simulink model "AreaCoverageTestHarness"  (R2016a)
settings: Solver=FixedStepDiscrete  StartTime=0.0  StopTime=6000  FixedStep=0.005  RelTol=1e-3
values from neighbouring files (symbols this model uses):
  BLOCK_SIZE = CAL_BLOCK_SIZE    [AreaCoverageCalib.m]    (also in room_V1.m = 20; room_V3.m = 20)
  EAST = 0    [AreaCoverageCalib.m]
  ERRVAL = 5    [AreaCoverageCalib.m]
  initXSim = 35    [AreaCoverageCalib.m]
  initYSim = 50    [AreaCoverageCalib.m]
  MAX_SPEED = 1000    [AreaCoverageCalib.m]
  MOTOR_HIGH = CAL_MOTOR_HIGH    [AreaCoverageCalib.m]
  MOTOR_LOW = CAL_MOTOR_LOW    [AreaCoverageCalib.m]
  NORTH = 270    [AreaCoverageCalib.m]
  PLOT_SAMPLE = 10    [AreaCoverageCalib.m]
  ROB_LENG = CAL_ROBO_LENG    [AreaCoverageCalib.m]
  ROB_WHEEL_R = .15    (= 0.15)    [AreaCoverageCalib.m]
  room = uint8(ones(side_size , side_size)*255)    [room_V1.m]    (also in room_V3.m)
  ROOM_SIDE_SIZE = CAL_ROOM_SIDE_SIZE    [AreaCoverageCalib.m]    (also in room_V1.m = 20; room_V3.m = 20)
  SAMPLE_TIME = 0.001    [AreaCoverageCalib.m]
  SOUTH = 90    [AreaCoverageCalib.m]
  STEP_SIZE = 5    [AreaCoverageCalib.m]
  WEST = 180    [AreaCoverageCalib.m]
undefined symbols (not defined in the file or in its folder): ROBO_LENG, sigbuilder_block
libraries: simulink x4
(part 1 of 2)
settings Model: Creator=oelkawok  LastModifiedBy=omaro

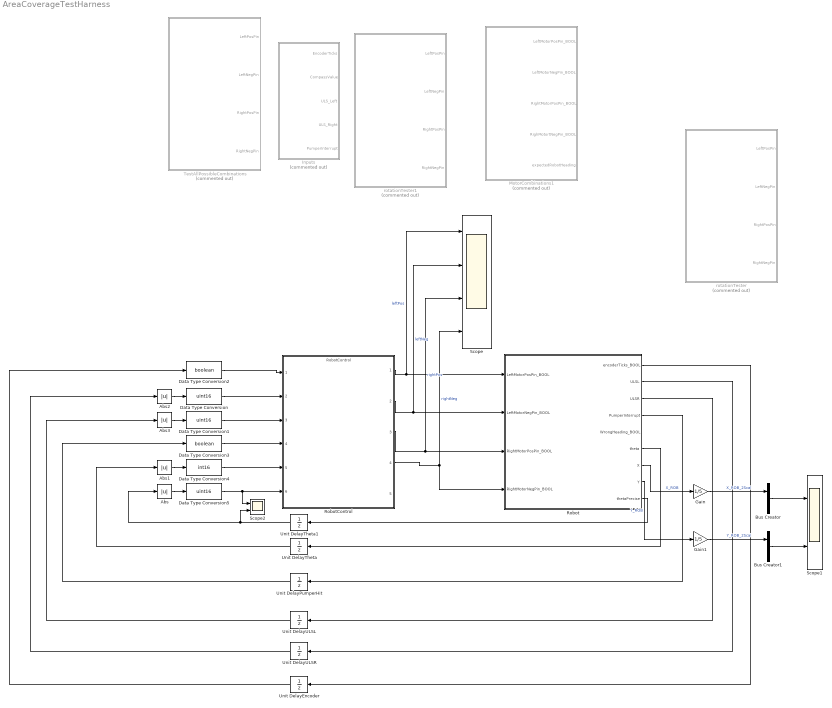
== system AreaCoverageTestHarness ==
  Abs{,1..3} (4 alike) : Abs
  Bus Creator : BusCreator  Inputs=2
  Bus Creator1 : BusCreator  Inputs=2
  Data Type Conversion : DataTypeConversion  OutDataTypeStr=uint16
  Data Type Conversion1 : DataTypeConversion  OutDataTypeStr=uint16
  Data Type Conversion2 : DataTypeConversion  OutDataTypeStr=boolean
  Data Type Conversion3 : DataTypeConversion  OutDataTypeStr=boolean
  Data Type Conversion4 : DataTypeConversion  OutDataTypeStr=int16
  Data Type Conversion5 : DataTypeConversion  OutDataTypeStr=uint16
  Gain : Gain  Gain=1/5  OutDataTypeStr=Inherit: Inherit via back propagation
  Gain1 : Gain  Gain=1/5  OutDataTypeStr=Inherit: Inherit via back propagation
  Inputs : Subsystem  Tag=STV Subsys  Commented=on  LoadFcn=sigbuilder_block('load');  StartFcn=sigbuilder_block('start');  StopFcn=sigbuilder_block('stop');  ClipboardFcn=sigbuilder_block('clipboard');  mask(Sigbuilder block){}
      mask help: Simulink:masks:SigbuilderBlock_MD
      mask init:
      | if ~strcmp(get_param(bdroot(gcbh),'SimulationStatus'),'stopped') tuvar = sigbuilder_block('maskInit'); end
      settings: CopyFcn=sigbuilder_block('copy');  DeleteFcn=sigbuilder_block('delete');  ModelCloseFcn=sigbuilder_block('modelClose');  PreSaveFcn=sigbuilder_block('preSave');  PauseFcn=sigbuilder_block('pause');  ContinueFcn=sigbuilder_block('continue');  NameChangeFcn=sigbuilder_block('namechange');  OpenFcn=sigbuilder_block('open',[211.2 103.8 550.8 400.2 ]);  CloseFcn=sigbuilder_block('close');
      mask Display: plot(0, 0, 100, 100,[2, 2, 32, 32, 2], [68, 8, 8, 68, 68],[32, 2], [38, 38], [32, 19, 2],[53, 60, 44], [32, 17, 17, 2],[16, 16, 31, 31]);txt = getActiveGroup(gcbh);text(2, 100, txt,'verticalAlignment', 'top');
  MotorCombinations1 : Subsystem  Commented=on
  Robot : Subsystem
  RobotControl : ModelReference  ModelNameDialog=RobotControl  SimulationMode=Normal  ModelReferenceVersion=1.370
  Scope : Scope  NumInputPorts=4
  Scope1 : Scope  NumInputPorts=2
  Scope2 : Scope  NumInputPorts=2
  TestAllPossibleCombinations : Subsystem  Tag=STV Subsys  Commented=on  LoadFcn=sigbuilder_block('load');  StartFcn=sigbuilder_block('start');  StopFcn=sigbuilder_block('stop');  ClipboardFcn=sigbuilder_block('clipboard');  mask(Sigbuilder block){}
      mask help: Simulink:masks:SigbuilderBlock_MD
      mask init:
      | if ~strcmp(get_param(bdroot(gcbh),'SimulationStatus'),'stopped') tuvar = sigbuilder_block('maskInit'); end
      settings: CopyFcn=sigbuilder_block('copy');  DeleteFcn=sigbuilder_block('delete');  ModelCloseFcn=sigbuilder_block('modelClose');  PreSaveFcn=sigbuilder_block('preSave');  PauseFcn=sigbuilder_block('pause');  ContinueFcn=sigbuilder_block('continue');  NameChangeFcn=sigbuilder_block('namechange');  OpenFcn=sigbuilder_block('open',[5.4 28.8 1141.2 525 ]);  CloseFcn=sigbuilder_block('close');
      mask Display: plot(0, 0, 100, 100,[2, 2, 32, 32, 2], [68, 8, 8, 68, 68],[32, 2], [38, 38], [32, 19, 2],[53, 60, 44], [32, 17, 17, 2],[16, 16, 31, 31]);txt = getActiveGroup(gcbh);text(2, 100, txt,'verticalAlignment', 'top');
  Unit DelayEncoder : UnitDelay  SampleTime=-1
  Unit DelayPumperHit : UnitDelay  SampleTime=-1
  Unit DelayTheta : UnitDelay  InitialCondition=NORTH  SampleTime=-1
      settings: AttributesFormatString=%<InitialCondition>
  Unit DelayTheta1 : UnitDelay  InitialCondition=NORTH*100  SampleTime=-1
      settings: AttributesFormatString=%<InitialCondition>
  Unit DelayULSL : UnitDelay  SampleTime=-1
  Unit DelayULSR : UnitDelay  SampleTime=-1
  rotationTester : Subsystem  Tag=STV Subsys  Commented=on  LoadFcn=sigbuilder_block('load');  StartFcn=sigbuilder_block('start');  StopFcn=sigbuilder_block('stop');  ClipboardFcn=sigbuilder_block('clipboard');  mask(Sigbuilder block){}
      mask help: Simulink:masks:SigbuilderBlock_MD
      mask init:
      | if ~strcmp(get_param(bdroot(gcbh),'SimulationStatus'),'stopped') tuvar = sigbuilder_block('maskInit'); end
      settings: CopyFcn=sigbuilder_block('copy');  DeleteFcn=sigbuilder_block('delete');  ModelCloseFcn=sigbuilder_block('modelClose');  PreSaveFcn=sigbuilder_block('preSave');  PauseFcn=sigbuilder_block('pause');  ContinueFcn=sigbuilder_block('continue');  NameChangeFcn=sigbuilder_block('namechange');  OpenFcn=sigbuilder_block('open',[6 28.2 1012.8 484.8 ]);  CloseFcn=sigbuilder_block('close');
      mask Display: plot(0, 0, 100, 100,[2, 2, 32, 32, 2], [68, 8, 8, 68, 68],[32, 2], [38, 38], [32, 19, 2],[53, 60, 44], [32, 17, 17, 2],[16, 16, 31, 31]);txt = getActiveGroup(gcbh);text(2, 100, txt,'verticalAlignment', 'top');
  rotationTester1 : Subsystem  Tag=STV Subsys  Commented=on  LoadFcn=sigbuilder_block('load');  StartFcn=sigbuilder_block('start');  StopFcn=sigbuilder_block('stop');  ClipboardFcn=sigbuilder_block('clipboard');  mask(Sigbuilder block){}
      mask help: Simulink:masks:SigbuilderBlock_MD
      mask init:
      | if ~strcmp(get_param(bdroot(gcbh),'SimulationStatus'),'stopped') tuvar = sigbuilder_block('maskInit'); end
      settings: CopyFcn=sigbuilder_block('copy');  DeleteFcn=sigbuilder_block('delete');  ModelCloseFcn=sigbuilder_block('modelClose');  PreSaveFcn=sigbuilder_block('preSave');  PauseFcn=sigbuilder_block('pause');  ContinueFcn=sigbuilder_block('continue');  NameChangeFcn=sigbuilder_block('namechange');  OpenFcn=sigbuilder_block('open',[5.4 28.8 1141.2 525 ]);  CloseFcn=sigbuilder_block('close');
      mask Display: plot(0, 0, 100, 100,[2, 2, 32, 32, 2], [68, 8, 8, 68, 68],[32, 2], [38, 38], [32, 19, 2],[53, 60, 44], [32, 17, 17, 2],[16, 16, 31, 31]);txt = getActiveGroup(gcbh);text(2, 100, txt,'verticalAlignment', 'top');
  wires:
  Data Type Conversion/1 -> RobotControl/2
  Data Type Conversion2/1 -> RobotControl/1
  Data Type Conversion1/1 -> RobotControl/3
  Data Type Conversion3/1 -> RobotControl/4
  Robot/1(encoderTicks_BOOL) -> Unit DelayEncoder/1
  Robot/3(ULSR) -> Unit DelayULSL/1
  Robot/4(PumperInterrupt) -> Unit DelayPumperHit/1
  Robot/2(ULSL) -> Unit DelayULSR/1
  Unit DelayPumperHit/1 -> Data Type Conversion3/1
  Unit DelayULSL/1 -> Abs3/1
  Unit DelayULSR/1 -> Abs2/1
  Unit DelayEncoder/1 -> Data Type Conversion2/1
  RobotControl/1 -> Scope/1, Robot/1(LeftMotorPosPin_BOOL)  "leftPos"
  RobotControl/2 -> Scope/2, Robot/2(LeftMotorNegPin_BOOL)  "leftNeg"
  RobotControl/3 -> Scope/3, Robot/3(RightMotorPosPin_BOOL)  "rightPos"
  RobotControl/4 -> Robot/4(RightMotorNegPin_BOOL), Scope/4  "rightNeg"
  Robot/6(theta) -> Unit DelayTheta/1
  Unit DelayTheta/1 -> Abs1/1
  Data Type Conversion4/1 -> RobotControl/5
  Robot/9(thetaPrecise) -> Unit DelayTheta1/1
  Data Type Conversion5/1 -> Scope2/1, RobotControl/6
  Unit DelayTheta1/1 -> Scope2/2, Abs/1
  Robot/7(X) -> Gain/1  "X_ROB"
  Robot/8(Y) -> Gain1/1  "Y_ROB"
  Bus Creator/1 -> Scope1/1
  Bus Creator1/1 -> Scope1/2
  Gain/1 -> Bus Creator/1  "X_ROB_2Scal"
  Gain1/1 -> Bus Creator1/1  "Y_ROB_2Scal"
  Abs/1 -> Data Type Conversion5/1
  Abs1/1 -> Data Type Conversion4/1
  Abs2/1 -> Data Type Conversion/1
  Abs3/1 -> Data Type Conversion1/1

== system AreaCoverageTestHarness/Inputs ==
  Demux : Demux  Tag=STV Demux  Outputs=5
  FromWs : FromWorkspace  Tag=STV FromWs  VariableName=tuvar  SampleTime=0
      SigBuilderData=|
      | common.afterFinalStr = 'Extrapolate'
      | common.sampleTime = 0
      | dataSet.timeRange = [0 10]
      | dataSet.name = 'Group 1'
      | sbobj.Groups.Name = 'Group 1'
      | sbobj.Groups.Signals(1).Name = 'EncoderTicks'
      | sbobj.Groups.Signals(1).XData = [0 4 4 6 6 10]
      | sbobj.Groups.Signals(1).YData = [0 0 1 1 0 0]
      | sbobj.Groups.Signals(2).Name = 'CompassValue'
      | sbobj.Groups.Signals(2).XData = [0 4 4 6 6 10]
      | sbobj.Groups.Signals(2).YData = [0 0 1 1 0 0]
      | sbobj.Groups.Signals(3).Name = 'ULS_Left'
      | sbobj.Groups.Signals(3).XData = [0 4 4 6 6 10]
      | sbobj.Groups.Signals(3).YData = [0 0 1 1 0 0]
      | sbobj.Groups.Signals(4).Name = 'ULS_Right'
      | sbobj.Groups.Signals(4).XData = [0 4 4 6 6 10]
      | sbobj.Groups.Signals(4).YData = [0 0 1 1 0 0]
      | sbobj.Groups.Signals(5).Name = 'PumperInterrupt'
      | sbobj.Groups.Signals(5).XData = [0 4 4 6 6 10]
      | sbobj.Groups.Signals(5).YData = [0 0 1 1 0 0]
  EncoderTicks : Outport  Tag=STV Outport
  CompassValue : Outport  Tag=STV Outport  Port=2
  ULS_Left : Outport  Tag=STV Outport  Port=3
  ULS_Right : Outport  Tag=STV Outport  Port=4
  PumperInterrupt : Outport  Tag=STV Outport  Port=5
  wires:
  Demux/1 -> EncoderTicks/1
  FromWs/1 -> Demux/1
  Demux/2 -> CompassValue/1
  Demux/3 -> ULS_Left/1
  Demux/4 -> ULS_Right/1
  Demux/5 -> PumperInterrupt/1

== system AreaCoverageTestHarness/MotorCombinations1 ==
  Signal Builder : Subsystem  Tag=STV Subsys  LoadFcn=sigbuilder_block('load');  StartFcn=sigbuilder_block('start');  StopFcn=sigbuilder_block('stop');  ClipboardFcn=sigbuilder_block('clipboard');  mask(Sigbuilder block){}
      mask help: Simulink:masks:SigbuilderBlock_MD
      mask init:
      | if ~strcmp(get_param(bdroot(gcbh),'SimulationStatus'),'stopped') tuvar = sigbuilder_block('maskInit'); end
      settings: CopyFcn=sigbuilder_block('copy');  DeleteFcn=sigbuilder_block('delete');  ModelCloseFcn=sigbuilder_block('modelClose');  PreSaveFcn=sigbuilder_block('preSave');  PauseFcn=sigbuilder_block('pause');  ContinueFcn=sigbuilder_block('continue');  NameChangeFcn=sigbuilder_block('namechange');  OpenFcn=sigbuilder_block('open',[0 28.8 1152 564 ]);  CloseFcn=sigbuilder_block('close');
      mask Display: plot(0, 0, 100, 100,[2, 2, 32, 32, 2], [68, 8, 8, 68, 68],[32, 2], [38, 38], [32, 19, 2],[53, 60, 44], [32, 17, 17, 2],[16, 16, 31, 31]);txt = getActiveGroup(gcbh);text(2, 100, txt,'verticalAlignment', 'top');
  LeftMotorPosPin_BOOL : Outport
  LeftMotorNegPin_BOOL : Outport  Port=2
  RightMotorPosPin_BOOL : Outport  Port=3
  RighMotortNegPin_BOOL : Outport  Port=4
  expectedRobotHeading : Outport  Port=5
  wires:
  Signal Builder/5(expectedRobotHeading) -> expectedRobotHeading/1
  Signal Builder/1(LeftPosPin) -> LeftMotorPosPin_BOOL/1  "LeftMotorPosPin_BOOL"
  Signal Builder/2(LeftNegPin) -> LeftMotorNegPin_BOOL/1  "LeftMotorNegPin_BOOL"
  Signal Builder/3(RightPosPin) -> RightMotorPosPin_BOOL/1  "RightMotorPosPin_BOOL"
  Signal Builder/4(RightNegPin) -> RighMotortNegPin_BOOL/1  "RighMotortNegPin_BOOL"

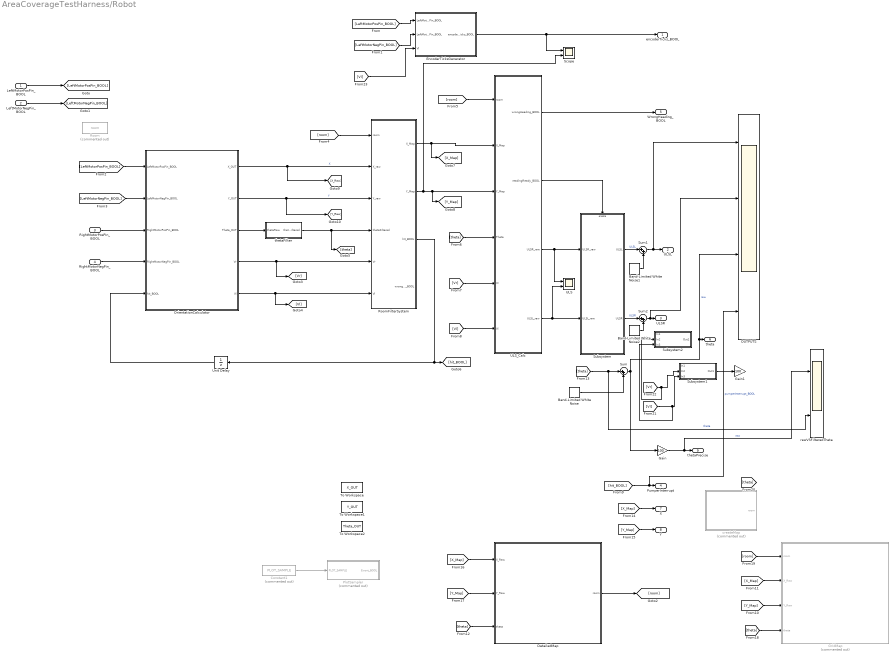
== system AreaCoverageTestHarness/Robot ==
  LeftMotorPosPin_BOOL : Inport
  LeftMotorNegPin_BOOL : Inport  Port=2
  RightMotorPosPin_BOOL : Inport  Port=3
  RightMotorNegPin_BOOL : Inport  Port=4
  Band-Limited White Noise : simulink/Sources/Band-Limited White Noise  Cov=[0.001]  Ts=0.005  seed=[23]
  Band-Limited White Noise1 : simulink/Sources/Band-Limited White Noise  Cov=[0.001]  Ts=0.005  seed=[23]
  Band-Limited White Noise2 : simulink/Sources/Band-Limited White Noise  Cov=[0.001]  Ts=0.005  seed=[23]
  Constant1 : Constant  Commented=on  Value=PLOT_SAMPLE
  DetailedMap : Subsystem
  EncoderTicksGenerator : Subsystem
  Gain : Gain  Gain=100
  Gain1 : Gain  Gain=100
  GridMap : Subsystem  Commented=on
  OUTPUTS : Scope  NumInputPorts=4
  OrientationCalculator : Subsystem
  PlotSampler : Stateflow chart  Commented=on  TreatAsAtomicUnit=on
  Room : Constant  Commented=on  Value=room
  RoomFilterSystem : Subsystem
  Scope : Scope  NumInputPorts=2
  Subsystem : Subsystem
  Subsystem1 : Subsystem
  Subsystem2 : Subsystem
  Sum : Sum  Inputs=|++
  Sum1 : Sum  Inputs=|++
  Sum2 : Sum  Inputs=|++
  To Workspace : ToWorkspace  VariableName=X_OUT  SaveFormat=Timeseries  SampleTime=-1
  To Workspace1 : ToWorkspace  VariableName=Y_OUT  SaveFormat=Timeseries  SampleTime=-1
  To Workspace2 : ToWorkspace  VariableName=Theta_OUT  SaveFormat=Timeseries  SampleTime=-1
  ULS : Scope  NumInputPorts=2
  ULS_Calc : Subsystem
  Unit Delay : UnitDelay  SampleTime=-1
      settings: AttributesFormatString=%<InitialCondition>
  createMap : Subsystem  Commented=on
  rawVSFilteredTheta : Scope  NumInputPorts=2
  thetaFilter : Subsystem
  encoderTicks_BOOL : Outport
  ULSL : Outport  Port=2
  ULSR : Outport  Port=3
  PumperInterrupt : Outport  Port=4
  WrongHeading_BOOL : Outport  Port=5
  theta : Outport  Port=6
  X : Outport  Port=7
  Y : Outport  Port=8
  thetaPrecise : Outport  Port=9
  wires:
  LeftMotorPosPin_BOOL/1 -> [LeftMotorPosPin_BOOL]
  LeftMotorNegPin_BOOL/1 -> [LeftMotorNegPin_BOOL]
  [LeftMotorNegPin_BOOL] -> EncoderTicksGenerator/2(LeftMotorNegPin_BOOL)
  [LeftMotorPosPin_BOOL] -> EncoderTicksGenerator/1(LeftMotorPosPin_BOOL)
  EncoderTicksGenerator/1(encoderTicks_BOOL) -> Scope/1, encoderTicks_BOOL/1
  [LeftMotorNegPin_BOOL] -> OrientationCalculator/2(LeftMotorNegPin_BOOL)
  [LeftMotorPosPin_BOOL] -> OrientationCalculator/1(LeftMotorPosPin_BOOL)
  RightMotorNegPin_BOOL/1 -> OrientationCalculator/4(RightMotorNegPin_BOOL)
  RightMotorPosPin_BOOL/1 -> OrientationCalculator/3(RightMotorPosPin_BOOL)
  OrientationCalculator/3(Theta_OUT) -> thetaFilter/1(thetaRaw)
  thetaFilter/1(thetaFiltered) -> RoomFilterSystem/4(thetaFiltered), [theta]
  OrientationCalculator/5(Vl) -> [Vl], RoomFilterSystem/6(Vl)
  OrientationCalculator/4(Vr) -> [Vr], RoomFilterSystem/5(Vr)
  RoomFilterSystem/3(hit_BOOL) -> [hit_BOOL], Unit Delay/1
  Unit Delay/1 -> OrientationCalculator/5(hit_BOOL)
  [room] -> RoomFilterSystem/1(room)
  [room] -> ULS_Calc/1(room)
  [theta] -> ULS_Calc/4(Theta)
  [Vr] -> ULS_Calc/5(Vr)
  [Vl] -> ULS_Calc/6(Vl)
  ULS_Calc/2(readingReady_BOOL) -> Subsystem/Enable
  ULS_Calc/4(ULSL_raw) -> ULS/2, Subsystem/2(ULSL_raw)
  ULS_Calc/3(ULSR_raw) -> ULS/1, Subsystem/1(ULSR_raw)
  [hit_BOOL] -> OUTPUTS/4, PumperInterrupt/1  "pumperInterrupt_BOOL"
  ULS_Calc/1(wrongHeading_BOOL) -> WrongHeading_BOOL/1
  Constant1/1 -> PlotSampler/1(PLOT_SAMPLE)
  RoomFilterSystem/2(Y_Map) -> ULS_Calc/3(Y_Map), [Y_Map], Scope/2
  RoomFilterSystem/1(X_Map) -> [X_Map], ULS_Calc/2(X_Map)
  [Y_Map] -> Y/1
  [X_Map] -> X/1
  OrientationCalculator/1(X_OUT) -> [X_Raw], RoomFilterSystem/2(X_raw)  "X"
  OrientationCalculator/2(Y_OUT) -> [Y_Raw], RoomFilterSystem/3(Y_raw)  "Y"
  [X_Map] -> DetailedMap/1(X_Raw)
  [Y_Map] -> DetailedMap/2(Y_Raw)
  [theta] -> DetailedMap/3(theta)
  [X_Map] -> GridMap/2(X_Raw)
  [Y_Map] -> GridMap/3(Y_Raw)
  [theta] -> GridMap/4(theta)
  [room] -> GridMap/1(room)
  DetailedMap/1(room) -> [room]
  Gain/1 -> rawVSFilteredTheta/1, thetaPrecise/1  "raw"
  [theta] -> rawVSFilteredTheta/2, Sum/1  "theta"
  Subsystem1/1(Out1) -> Gain1/1
  [Vr] -> Subsystem2/2(In2), Subsystem1/2(In2)
  [Vl] -> Subsystem2/3(In3), Subsystem1/3(In3)
  Sum/1 -> OUTPUTS/3, theta/1, Gain/1  "raw"
  [Vl] -> EncoderTicksGenerator/3(Vl)
  Band-Limited White Noise/1 -> Sum/2
  Subsystem/1(ULSL) -> Sum1/1  "ULSL"
  Sum1/1 -> OUTPUTS/1, ULSL/1
  Band-Limited White Noise1/1 -> Sum1/2
  Sum2/1 -> OUTPUTS/2, ULSR/1
  Band-Limited White Noise2/1 -> Sum2/2
  Subsystem/2(ULSR) -> Sum2/1  "ULSR"

== system AreaCoverageTestHarness/TestAllPossibleCombinations ==
  Demux : Demux  Tag=STV Demux
  FromWs : FromWorkspace  Tag=STV FromWs  VariableName=tuvar  SampleTime=0
      SigBuilderData=|
      | common.afterFinalStr = 'Extrapolate'
      | common.sampleTime = 0
      | dataSet.timeRange = [0 16]
      | dataSet.name = 'Group 1'
      | sbobj.Groups.Name = 'Group 1'
      | sbobj.Groups.Signals(1).Name = 'LeftPosPin'
      | sbobj.Groups.Signals(1).XData = [0 8 8 13.8 16]
      | sbobj.Groups.Signals(1).YData = [0 0 1 1 1]
      | sbobj.Groups.Signals(2).Name = 'LeftNegPin'
      | sbobj.Groups.Signals(2).XData = [0 1 2 4 4 8 8 12 12 16]
      | sbobj.Groups.Signals(2).YData = [0 0 0 0 1 1 0 0 1 1]
      | sbobj.Groups.Signals(3).Name = 'RightPosPin'
      | sbobj.Groups.Signals(3).XData = [0 1 2 4 4 6 8 8 10 10 12 12 14 14 16]
      | sbobj.Groups.Signals(3).YData = [0 0 0 0 1 1 1 0 0 1 1 0 0 1 1]
      | sbobj.Groups.Signals(4).Name = 'RightNegPin'
      | sbobj.Groups.Signals(4).XData = [0 1 1 3.08 3.08 8 11 11 12 12 13 13 14 14 15 15 16]
      | sbobj.Groups.Signals(4).YData = [0 0 1 1 0 0 0 1 1 0 0 1 1 0 0 1 1]
      | sbobj.Groups.TimeRange = [0 16]
  LeftPosPin : Outport  Tag=STV Outport
  LeftNegPin : Outport  Tag=STV Outport  Port=2
  RightPosPin : Outport  Tag=STV Outport  Port=3
  RightNegPin : Outport  Tag=STV Outport  Port=4
  wires:
  Demux/1 -> LeftPosPin/1
  FromWs/1 -> Demux/1
  Demux/2 -> LeftNegPin/1
  Demux/3 -> RightPosPin/1
  Demux/4 -> RightNegPin/1

== system AreaCoverageTestHarness/rotationTester ==
  Demux : Demux  Tag=STV Demux
  FromWs : FromWorkspace  Tag=STV FromWs  VariableName=tuvar  SampleTime=0
      SigBuilderData=|
      | common.afterFinalStr = 'Extrapolate'
      | common.sampleTime = 0
      | dataSet.timeRange = [0 16]
      | dataSet.name = 'Group 1'
      | sbobj.Groups.Name = 'Group 1'
      | sbobj.Groups.Signals(1).Name = 'LeftPosPin'
      | sbobj.Groups.Signals(1).XData = [0 2 3.35 8 8 12.16 12.16 16]
      | sbobj.Groups.Signals(1).YData = [1 1 1 1 0 0 1 1]
      | sbobj.Groups.Signals(2).Name = 'LeftNegPin'
      | sbobj.Groups.Signals(2).XData = [0 1 2.18 10 10 12 12 16]
      | sbobj.Groups.Signals(2).YData = [0 0 0 0 1 1 0 0]
      | sbobj.Groups.Signals(3).Name = 'RightPosPin'
      | sbobj.Groups.Signals(3).XData = [0 1 2 8 12.28 12.28 16]
      | sbobj.Groups.Signals(3).YData = [0 0 0 0 0 1 1]
      | sbobj.Groups.Signals(4).Name = 'RightNegPin'
      | sbobj.Groups.Signals(4).XData = [0 2 3.35 8 8 10 10 12 12 16]
      | sbobj.Groups.Signals(4).YData = [1 1 1 1 0 0 1 1 0 0]
      | sbobj.Groups.TimeRange = [0 16]
  LeftPosPin : Outport  Tag=STV Outport
  LeftNegPin : Outport  Tag=STV Outport  Port=2
  RightPosPin : Outport  Tag=STV Outport  Port=3
  RightNegPin : Outport  Tag=STV Outport  Port=4
  wires:
  Demux/4 -> RightNegPin/1
  Demux/3 -> RightPosPin/1
  Demux/2 -> LeftNegPin/1
  FromWs/1 -> Demux/1
  Demux/1 -> LeftPosPin/1

== system AreaCoverageTestHarness/rotationTester1 ==
  Demux : Demux  Tag=STV Demux
  FromWs : FromWorkspace  Tag=STV FromWs  VariableName=tuvar  SampleTime=0
      SigBuilderData=|
      | common.afterFinalStr = 'Extrapolate'
      | common.sampleTime = 0
      | dataSet.timeRange = [0 16]
      | dataSet.name = 'Group 1'
      | sbobj.Groups.Name = 'Group 1'
      | sbobj.Groups.Signals(1).Name = 'LeftPosPin'
      | sbobj.Groups.Signals(1).XData = [0 2.14 2.14 13.8 16]
      | sbobj.Groups.Signals(1).YData = [0 0 1 1 1]
      | sbobj.Groups.Signals(2).Name = 'LeftNegPin'
      | sbobj.Groups.Signals(2).XData = [0 1 1 2.08 2.08 12 16]
      | sbobj.Groups.Signals(2).YData = [0 0 1 1 0 0 0]
      | sbobj.Groups.Signals(3).Name = 'RightPosPin'
      | sbobj.Groups.Signals(3).XData = [0 1 2.08 2.08 13.18 14 14 16]
      | sbobj.Groups.Signals(3).YData = [0 0 0 1 1 1 0 0]
      | sbobj.Groups.Signals(4).Name = 'RightNegPin'
      | sbobj.Groups.Signals(4).XData = [0 1 1 8 11 12 13 14 15 16]
      | sbobj.Groups.Signals(4).YData = [0 0 1 1 1 1 1 1 1 1]
      | sbobj.Groups.TimeRange = [0 16]
  LeftPosPin : Outport  Tag=STV Outport
  LeftNegPin : Outport  Tag=STV Outport  Port=2
  RightPosPin : Outport  Tag=STV Outport  Port=3
  RightNegPin : Outport  Tag=STV Outport  Port=4
  wires:
  Demux/1 -> LeftPosPin/1
  FromWs/1 -> Demux/1
  Demux/2 -> LeftNegPin/1
  Demux/3 -> RightPosPin/1
  Demux/4 -> RightNegPin/1

== system AreaCoverageTestHarness/MotorCombinations1/Signal Builder ==
  Demux : Demux  Tag=STV Demux  Outputs=5
  FromWs : FromWorkspace  Tag=STV FromWs  VariableName=tuvar  SampleTime=0
      SigBuilderData=|
      | common.afterFinalStr = 'Extrapolate'
      | common.sampleTime = 0
      | dataSet.timeRange = [0 16]
      | dataSet.name = 'Group 1'
      | sbobj.Groups.Name = 'Group 1'
      | sbobj.Groups.Signals(1).Name = 'LeftPosPin'
      | sbobj.Groups.Signals(1).XData = [0 8 8 13.8 16]
      | sbobj.Groups.Signals(1).YData = [0 0 1 1 1]
      | sbobj.Groups.Signals(2).Name = 'LeftNegPin'
      | sbobj.Groups.Signals(2).XData = [0 1 2 4 4 8 8 12 12 16]
      | sbobj.Groups.Signals(2).YData = [0 0 0 0 1 1 0 0 1 1]
      | sbobj.Groups.Signals(3).Name = 'RightPosPin'
      | sbobj.Groups.Signals(3).XData = [0 1 2 2 4 4 6 6 8 8 10 10 12 12 14 14 16]
      | sbobj.Groups.Signals(3).YData = [0 0 0 1 1 0 0 1 1 0 0 1 1 0 0 1 1]
      | sbobj.Groups.Signals(4).Name = 'RightNegPin'
      | sbobj.Groups.Signals(4).XData = [0 1 1 2 2 3 3 4 4 5 5 6 6 7 7 8 8 9 9 10 10 11 11 12 12 13 13 14 14 15 15 16]
      | sbobj.Groups.Signals(4).YData = [0 0 1 1 0 0 1 1 0 0 1 1 0 0 1 1 0 0 1 1 0 0 1 1 0 0 1 1 0 0 1 1]
      | sbobj.Groups.Signals(5).Name = 'expectedRobotHeading'
      | sbobj.Groups.Signals(5).XData = [0 1 1 2 2 3 3 4 4 5 5 6 6 7 7 8 8 9 9 10 10 11 11 12 12 13 13 14 14 15 15 16]
      | sbobj.Groups.Signals(5).YData = [7 7 2 2 1 1 7 7 1 1 6 6 3 3 1 1 2 2 4 4 5 5 2 2 7 7 2 2 1 1 7 7]
      | sbobj.Groups.TimeRange = [0 16]
  LeftPosPin : Outport  Tag=STV Outport
  LeftNegPin : Outport  Tag=STV Outport  Port=2
  RightPosPin : Outport  Tag=STV Outport  Port=3
  RightNegPin : Outport  Tag=STV Outport  Port=4
  expectedRobotHeading : Outport  Tag=STV Outport  Port=5
  wires:
  Demux/5 -> expectedRobotHeading/1
  Demux/4 -> RightNegPin/1
  Demux/3 -> RightPosPin/1
  Demux/2 -> LeftNegPin/1
  FromWs/1 -> Demux/1
  Demux/1 -> LeftPosPin/1

== system AreaCoverageTestHarness/Robot/DetailedMap ==
  X_Raw : Inport
  Y_Raw : Inport  Port=2
  theta : Inport  Port=3
  Clock : Clock
  MATLAB Function : MATLAB Function  TreatAsAtomicUnit=on
  MapX_Y : Scope  NumInputPorts=2
  createMap : Subsystem  Variant=on  OverrideUsingVariant=Variant2
  room : Outport
  wires:
  theta/1 -> MATLAB Function/4(Theta)
  Clock/1 -> MATLAB Function/5(clock)
  createMap/1(room) -> room/1, MATLAB Function/1(room)
  X_Raw/1 -> MapX_Y/1, MATLAB Function/2(X)
  Y_Raw/1 -> MapX_Y/2, MATLAB Function/3(Y)

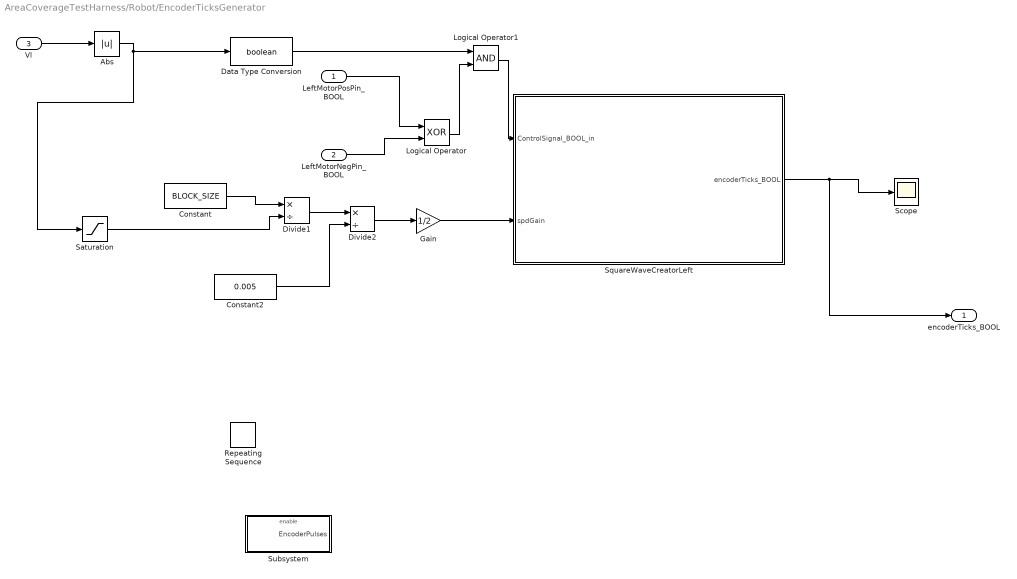
== system AreaCoverageTestHarness/Robot/EncoderTicksGenerator ==
  LeftMotorPosPin_BOOL : Inport
  LeftMotorNegPin_BOOL : Inport  Port=2
  Vl : Inport  Port=3
  Abs : Abs
  Constant : Constant  Value=BLOCK_SIZE
  Constant2 : Constant  Value=0.005
  Data Type Conversion : DataTypeConversion  OutDataTypeStr=boolean
  Divide1 : Product  Inputs=*/
  Divide2 : Product  Inputs=*/
  Gain : Gain  Gain=1/2
  Logical Operator : Logic  Operator=XOR  AllPortsSameDT=off  OutDataTypeStr=boolean
  Logical Operator1 : Logic  AllPortsSameDT=off  OutDataTypeStr=boolean
  Repeating Sequence : simulink/Sources/Repeating Sequence  rep_seq_t=[0 .5]  rep_seq_y=[0 0.5]
  Saturation : Saturate  UpperLimit=90000  LowerLimit=0.0001
  Scope : Scope
  SquareWaveCreatorLeft : Stateflow chart  TreatAsAtomicUnit=on
  Subsystem : Subsystem
  encoderTicks_BOOL : Outport
  wires:
  SquareWaveCreatorLeft/1(encoderTicks_BOOL) -> encoderTicks_BOOL/1, Scope/1
  Vl/1 -> Abs/1
  Constant/1 -> Divide1/1
  Divide1/1 -> Divide2/1
  Constant2/1 -> Divide2/2
  Divide2/1 -> Gain/1
  LeftMotorPosPin_BOOL/1 -> Logical Operator/1
  LeftMotorNegPin_BOOL/1 -> Logical Operator/2
  Logical Operator/1 -> Logical Operator1/2
  Abs/1 -> Data Type Conversion/1, Saturation/1
  Logical Operator1/1 -> SquareWaveCreatorLeft/1(ControlSignal_BOOL_in)
  Data Type Conversion/1 -> Logical Operator1/1
  Saturation/1 -> Divide1/2
  Gain/1 -> SquareWaveCreatorLeft/2(spdGain)

== system AreaCoverageTestHarness/Robot/GridMap ==
  room : Inport
  X_Raw : Inport  Port=2
  Y_Raw : Inport  Port=3
  theta : Inport  Port=4
  Clock : Clock
  MATLAB Function : MATLAB Function  TreatAsAtomicUnit=on
  MapX_Y : Scope  NumInputPorts=2
  wires:
  Y_Raw/1 -> MATLAB Function/3(Y), MapX_Y/2
  X_Raw/1 -> MATLAB Function/2(X), MapX_Y/1
  Clock/1 -> MATLAB Function/5(clock)
  theta/1 -> MATLAB Function/4(Theta)
  room/1 -> MATLAB Function/1(room)

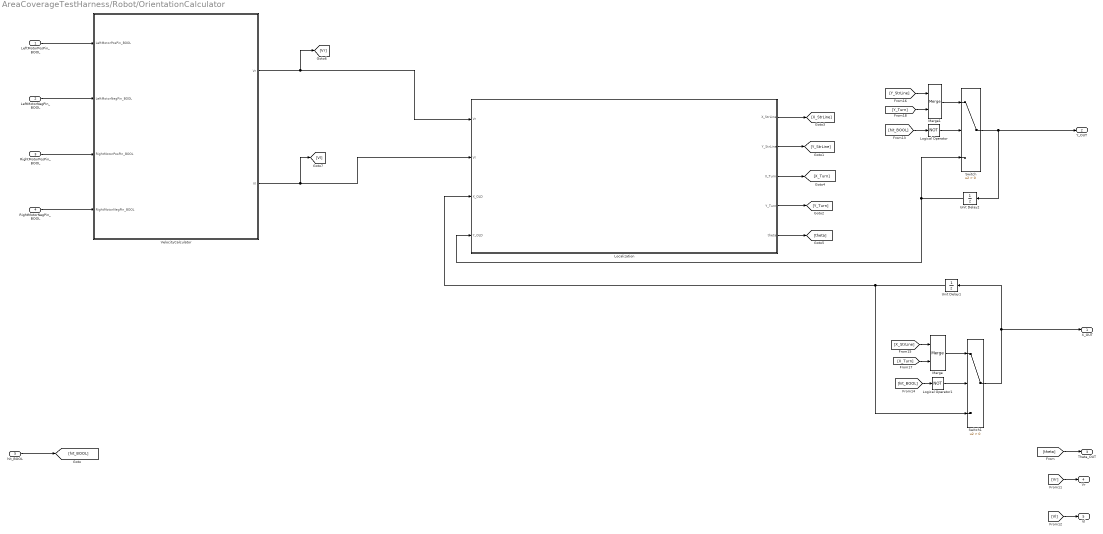
== system AreaCoverageTestHarness/Robot/OrientationCalculator ==
  LeftMotorPosPin_BOOL : Inport
  LeftMotorNegPin_BOOL : Inport  Port=2
  RightMotorPosPin_BOOL : Inport  Port=3
  RightMotorNegPin_BOOL : Inport  Port=4
  hit_BOOL : Inport  Port=5
  Localization : Subsystem
  Logical Operator : Logic  Operator=NOT  AllPortsSameDT=off  OutDataTypeStr=boolean
  Logical Operator1 : Logic  Operator=NOT  AllPortsSameDT=off  OutDataTypeStr=boolean
  Merge : Merge
  Merge1 : Merge
  Switch : Switch  Criteria=u2 > Threshold
  Switch1 : Switch  Criteria=u2 > Threshold
  Unit Delay1 : UnitDelay  InitialCondition=initXSim  SampleTime=-1
      settings: AttributesFormatString=%<InitialCondition>
  Unit Delay2 : UnitDelay  InitialCondition=initYSim  SampleTime=-1
      settings: AttributesFormatString=%<InitialCondition>
  VelocityCalculator : Subsystem
  X_OUT : Outport
  Y_OUT : Outport  Port=2
  Theta_OUT : Outport  Port=3
  Vr : Outport  Port=4
  Vl : Outport  Port=5
  wires:
  Unit Delay1/1 -> Localization/3(X_OLD), Switch1/3
  Unit Delay2/1 -> Switch/3, Localization/4(Y_OLD)
  Merge1/1 -> Switch/1
  [Vl] -> Vl/1
  [Vr] -> Vr/1
  hit_BOOL/1 -> [hit_BOOL]
  [hit_BOOL] -> Logical Operator/1
  Logical Operator/1 -> Switch/2
  Switch/1 -> Unit Delay2/1, Y_OUT/1
  [hit_BOOL] -> Logical Operator1/1
  Logical Operator1/1 -> Switch1/2
  Merge/1 -> Switch1/1
  Switch1/1 -> Unit Delay1/1, X_OUT/1
  LeftMotorPosPin_BOOL/1 -> VelocityCalculator/1(LeftMotorPosPin_BOOL)
  LeftMotorNegPin_BOOL/1 -> VelocityCalculator/2(LeftMotorNegPin_BOOL)
  RightMotorPosPin_BOOL/1 -> VelocityCalculator/3(RightMotorPosPin_BOOL)
  RightMotorNegPin_BOOL/1 -> VelocityCalculator/4(RightMotorNegPin_BOOL)
  VelocityCalculator/1(Vr) -> [Vr], Localization/1(Vr)
  VelocityCalculator/2(Vl) -> [Vl], Localization/2(Vl)
  [X_StrLine] -> Merge/1
  [Y_StrLine] -> Merge1/1
  [X_Turn] -> Merge/2
  [Y_Turn] -> Merge1/2
  Localization/2(Y_StrLine) -> [Y_StrLine]
  Localization/4(Y_Turn) -> [Y_Turn]
  Localization/1(X_StrLine) -> [X_StrLine]
  Localization/3(X_Turn) -> [X_Turn]
  Localization/5(theta) -> [theta]
  [theta] -> Theta_OUT/1

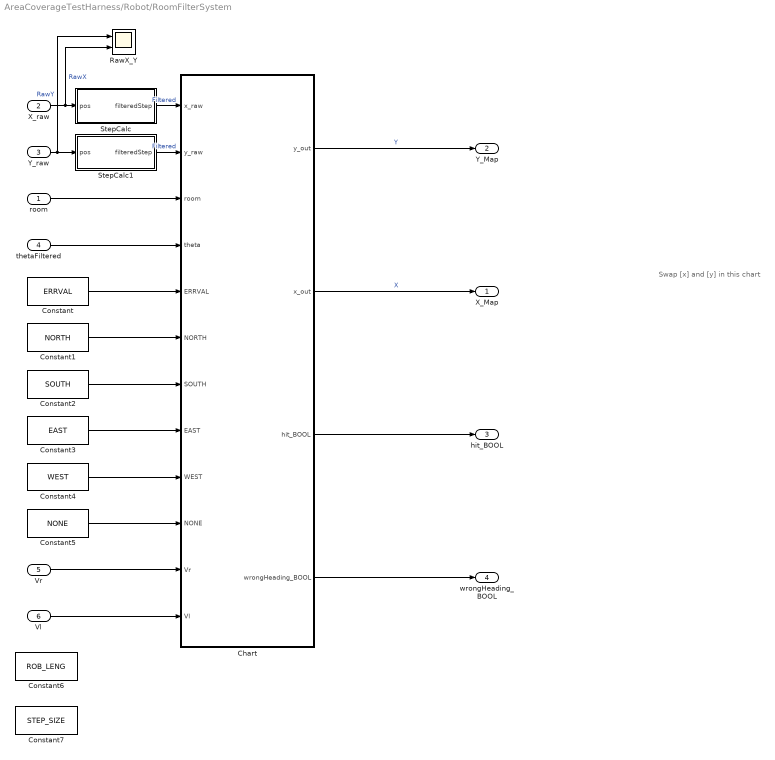
== system AreaCoverageTestHarness/Robot/RoomFilterSystem ==
  note: Swap [x] and [y] in this chart
  room : Inport
  X_raw : Inport  Port=2
  Y_raw : Inport  Port=3
  thetaFiltered : Inport  Port=4
  Vr : Inport  Port=5
  Vl : Inport  Port=6
  Chart : Stateflow chart  TreatAsAtomicUnit=on
  Constant : Constant  Value=ERRVAL
  Constant1 : Constant  Value=NORTH
  Constant2 : Constant  Value=SOUTH
  Constant3 : Constant  Value=EAST
  Constant4 : Constant  Value=WEST
  Constant5 : Constant  Value=NONE
  Constant6 : Constant  Value=ROB_LENG
  Constant7 : Constant  Value=STEP_SIZE
  RawX_Y : Scope  NumInputPorts=2
  StepCalc : Subsystem
  StepCalc1 : Subsystem
  X_Map : Outport
  Y_Map : Outport  Port=2
  hit_BOOL : Outport  Port=3
  wrongHeading_BOOL : Outport  Port=4
  wires:
  Y_raw/1 -> RawX_Y/1, StepCalc1/1(pos)  "RawY"
  room/1 -> Chart/3(room)
  Chart/1(y_out) -> Y_Map/1  "Y"
  Chart/2(x_out) -> X_Map/1  "X"
  thetaFiltered/1 -> Chart/4(theta)
  Constant/1 -> Chart/5(ERRVAL)
  Constant1/1 -> Chart/6(NORTH)
  Constant2/1 -> Chart/7(SOUTH)
  Constant5/1 -> Chart/10(NONE)
  Constant4/1 -> Chart/9(WEST)
  Constant3/1 -> Chart/8(EAST)
  Vr/1 -> Chart/11(Vr)
  Vl/1 -> Chart/12(Vl)
  Chart/3(hit_BOOL) -> hit_BOOL/1
  Chart/4(wrongHeading_BOOL) -> wrongHeading_BOOL/1
  StepCalc1/1(filteredStep) -> Chart/2(y_raw)  "Filtered"
  X_raw/1 -> RawX_Y/2, StepCalc/1(pos)  "RawX"
  StepCalc/1(filteredStep) -> Chart/1(x_raw)  "Filtered"

== system AreaCoverageTestHarness/Robot/Subsystem ==
  ULSR_raw : Inport
  ULSL_raw : Inport  Port=2
  Enable : EnablePort
      settings: AttributesFormatString=%<StatesWhenEnabling>
  Constant : Constant  Value=ROBO_LENG
  Constant1 : Constant  Value=ROBO_LENG
  Gain : Gain  Gain=BLOCK_SIZE/4
  Gain1 : Gain  Gain=BLOCK_SIZE/4
  Gain2 : Gain  Gain=0.5
  Gain3 : Gain  Gain=0.5
  Subtract : Sum  Inputs=+-
  Subtract1 : Sum  Inputs=+-
  ULSL : Outport
      settings: AttributesFormatString=%<OutputWhenDisabled>
  ULSR : Outport  Port=2
      settings: AttributesFormatString=%<OutputWhenDisabled>
  wires:
  ULSL_raw/1 -> Gain1/1
  ULSR_raw/1 -> Gain/1
  Gain1/1 -> Subtract1/1
  Gain/1 -> Subtract/1
  Subtract/1 -> ULSR/1
  Constant/1 -> Gain2/1
  Gain2/1 -> Subtract/2
  Constant1/1 -> Gain3/1
  Gain3/1 -> Subtract1/2
  Subtract1/1 -> ULSL/1

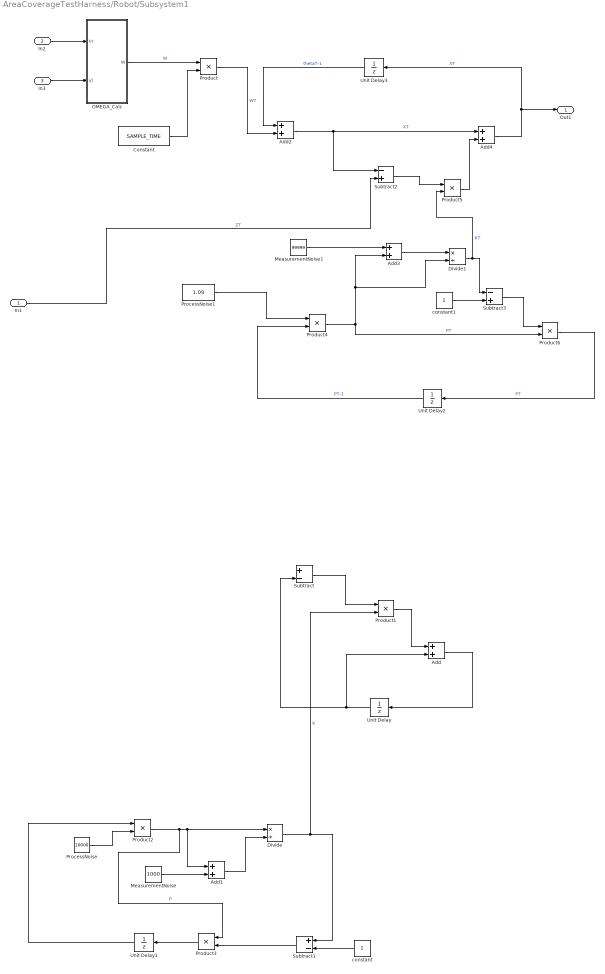
== system AreaCoverageTestHarness/Robot/Subsystem1 ==
  In1 : Inport
  In2 : Inport  Port=2
  In3 : Inport  Port=3
  Add{,1..4} (5 alike) : Sum
  Constant : Constant  Value=SAMPLE_TIME
  Divide : Product  Inputs=*/
  Divide1 : Product  Inputs=*/
  MeasurementNoise : Constant  Value=1000
  MeasurementNoise1 : Constant  Value=99999
  OMEGA_Calc : Subsystem
  ProcessNoise : Constant  Value=10000
  ProcessNoise1 : Constant  Value=1.09
  Product{,1..6} (7 alike) : Product
  Subtract : Sum  Inputs=+-
  Subtract1 : Sum  Inputs=+-
  Subtract2 : Sum  Inputs=-+
  Subtract3 : Sum  Inputs=-+
  Unit Delay : UnitDelay  SampleTime=-1
  Unit Delay1 : UnitDelay  InitialCondition=10  SampleTime=-1
  Unit Delay2 : UnitDelay  InitialCondition=1  SampleTime=-1
  Unit Delay3 : UnitDelay  InitialCondition=NORTH*100  SampleTime=-1
  constant : Constant
  constant1 : Constant
  Out1 : Outport
  wires:
  In3/1 -> OMEGA_Calc/2(Vl)
  In2/1 -> OMEGA_Calc/1(Vr)
  Constant/1 -> Product/2
  OMEGA_Calc/1(W) -> Product/1  "W"
  In1/1 -> Subtract2/2  "ZT"
  Add/1 -> Unit Delay/1
  Unit Delay/1 -> Add/2, Subtract/2
  Subtract/1 -> Product1/1
  Product1/1 -> Add/1
  ProcessNoise/1 -> Product2/2
  Product2/1 -> Divide/1, Add1/1, Product3/1  "P"
  MeasurementNoise/1 -> Add1/2
  Add1/1 -> Divide/2
  Divide/1 -> Subtract1/1, Product1/2  "K"
  Unit Delay1/1 -> Product2/1
  constant/1 -> Subtract1/2
  Subtract1/1 -> Product3/2
  Product3/1 -> Unit Delay1/1
  Product/1 -> Add2/2  "WT"
  Unit Delay3/1 -> Add2/1  "thetaT-1"
  ProcessNoise1/1 -> Product4/1
  Unit Delay2/1 -> Product4/2  "PT-1"
  Product4/1 -> Product6/2, Divide1/2, Add3/2  "PT"
  MeasurementNoise1/1 -> Add3/1
  Add3/1 -> Divide1/1
  Divide1/1 -> Subtract3/1, Product5/2  "KT"
  Add2/1 -> Subtract2/1, Add4/1  "XT"
  Subtract2/1 -> Product5/1
  constant1/1 -> Subtract3/2
  Subtract3/1 -> Product6/1
  Product6/1 -> Unit Delay2/1  "PT"
  Product5/1 -> Add4/2
  Add4/1 -> Out1/1, Unit Delay3/1  "XT"

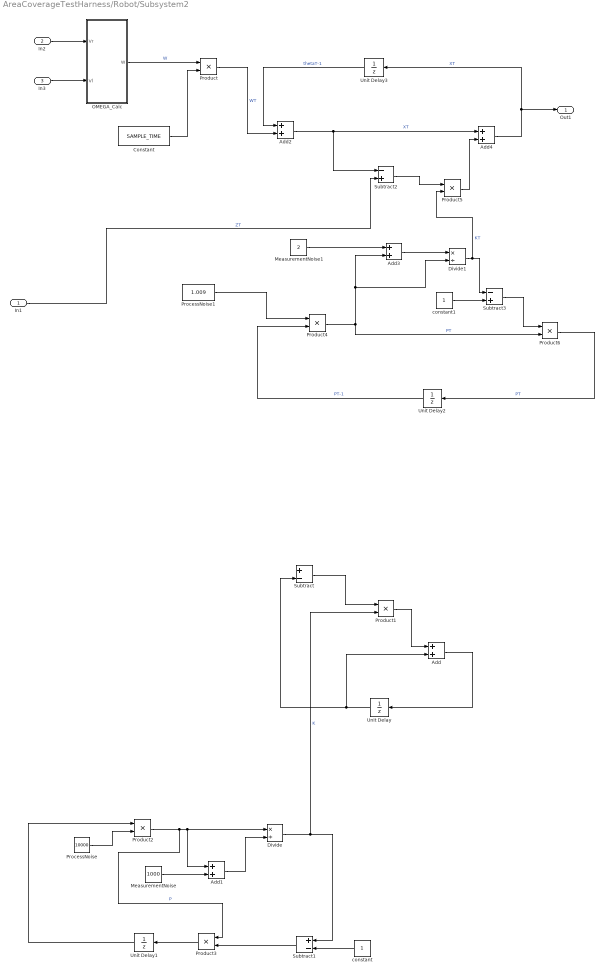
== system AreaCoverageTestHarness/Robot/Subsystem2 ==
  In1 : Inport
  In2 : Inport  Port=2
  In3 : Inport  Port=3
  Add{,1..4} (5 alike) : Sum
  Constant : Constant  Value=SAMPLE_TIME
  Divide : Product  Inputs=*/
  Divide1 : Product  Inputs=*/
  MeasurementNoise : Constant  Value=1000
  MeasurementNoise1 : Constant  Value=2
  OMEGA_Calc : Subsystem
  ProcessNoise : Constant  Value=10000
  ProcessNoise1 : Constant  Value=1.009
  Product{,1..6} (7 alike) : Product
  Subtract : Sum  Inputs=+-
  Subtract1 : Sum  Inputs=+-
  Subtract2 : Sum  Inputs=-+
  Subtract3 : Sum  Inputs=-+
  Unit Delay : UnitDelay  SampleTime=-1
  Unit Delay1 : UnitDelay  InitialCondition=10  SampleTime=-1
  Unit Delay2 : UnitDelay  InitialCondition=1  SampleTime=-1
  Unit Delay3 : UnitDelay  InitialCondition=NORTH  SampleTime=-1
  constant : Constant
  constant1 : Constant
  Out1 : Outport
  wires:
  Add4/1 -> Unit Delay3/1, Out1/1  "XT"
  Product5/1 -> Add4/2
  Product6/1 -> Unit Delay2/1  "PT"
  Subtract3/1 -> Product6/1
  constant1/1 -> Subtract3/2
  Subtract2/1 -> Product5/1
  Add2/1 -> Add4/1, Subtract2/1  "XT"
  Divide1/1 -> Product5/2, Subtract3/1  "KT"
  Add3/1 -> Divide1/1
  MeasurementNoise1/1 -> Add3/1
  Product4/1 -> Add3/2, Divide1/2, Product6/2  "PT"
  Unit Delay2/1 -> Product4/2  "PT-1"
  ProcessNoise1/1 -> Product4/1
  Unit Delay3/1 -> Add2/1  "thetaT-1"
  Product/1 -> Add2/2  "WT"
  Product3/1 -> Unit Delay1/1
  Subtract1/1 -> Product3/2
  constant/1 -> Subtract1/2
  Unit Delay1/1 -> Product2/1
  Divide/1 -> Product1/2, Subtract1/1  "K"
  Add1/1 -> Divide/2
  MeasurementNoise/1 -> Add1/2
  Product2/1 -> Product3/1, Add1/1, Divide/1  "P"
  ProcessNoise/1 -> Product2/2
  Product1/1 -> Add/1
  Subtract/1 -> Product1/1
  Unit Delay/1 -> Subtract/2, Add/2
  Add/1 -> Unit Delay/1
  In1/1 -> Subtract2/2  "ZT"
  OMEGA_Calc/1(W) -> Product/1  "W"
  Constant/1 -> Product/2
  In2/1 -> OMEGA_Calc/1(Vr)
  In3/1 -> OMEGA_Calc/2(Vl)

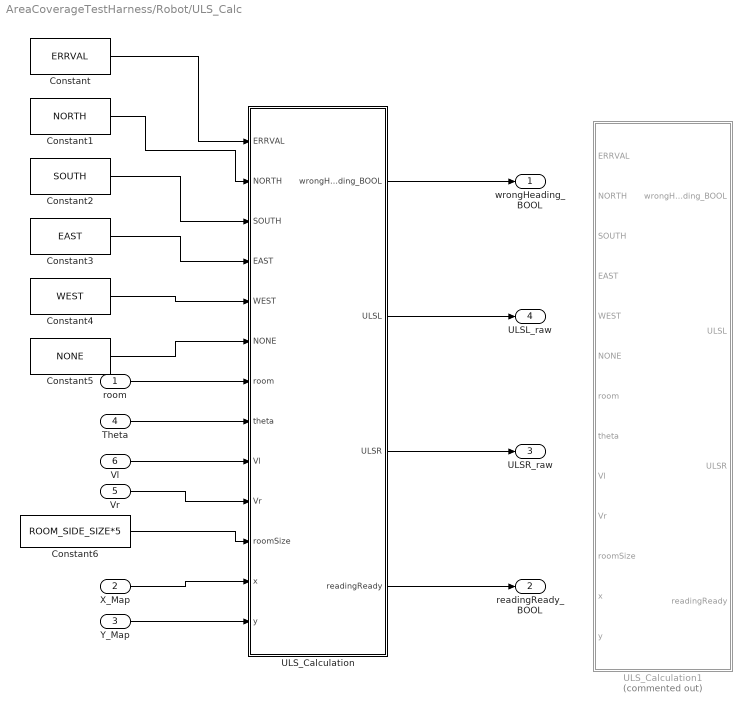
== system AreaCoverageTestHarness/Robot/ULS_Calc ==
  room : Inport
  X_Map : Inport  Port=2
  Y_Map : Inport  Port=3
  Theta : Inport  Port=4
  Vr : Inport  Port=5
  Vl : Inport  Port=6
  Constant : Constant  Value=ERRVAL
  Constant1 : Constant  Value=NORTH
  Constant2 : Constant  Value=SOUTH
  Constant3 : Constant  Value=EAST
  Constant4 : Constant  Value=WEST
  Constant5 : Constant  Value=NONE
  Constant6 : Constant  Value=ROOM_SIDE_SIZE*5
  ULS_Calculation : Stateflow chart  TreatAsAtomicUnit=on
  ULS_Calculation1 : Stateflow chart  Commented=on  TreatAsAtomicUnit=on
  wrongHeading_BOOL : Outport
  readingReady_BOOL : Outport  Port=2
  ULSR_raw : Outport  Port=3
  ULSL_raw : Outport  Port=4
  wires:
  X_Map/1 -> ULS_Calculation/12(x)
  Y_Map/1 -> ULS_Calculation/13(y)
  Theta/1 -> ULS_Calculation/8(theta)
  Constant4/1 -> ULS_Calculation/5(WEST)
  Constant5/1 -> ULS_Calculation/6(NONE)
  Constant3/1 -> ULS_Calculation/4(EAST)
  Constant2/1 -> ULS_Calculation/3(SOUTH)
  Constant1/1 -> ULS_Calculation/2(NORTH)
  Constant/1 -> ULS_Calculation/1(ERRVAL)
  room/1 -> ULS_Calculation/7(room)
  Constant6/1 -> ULS_Calculation/11(roomSize)
  Vl/1 -> ULS_Calculation/9(Vl)
  Vr/1 -> ULS_Calculation/10(Vr)
  ULS_Calculation/2(ULSL) -> ULSL_raw/1
  ULS_Calculation/3(ULSR) -> ULSR_raw/1
  ULS_Calculation/4(readingReady) -> readingReady_BOOL/1
  ULS_Calculation/1(wrongHeading_BOOL) -> wrongHeading_BOOL/1

== system AreaCoverageTestHarness/Robot/createMap ==
  MATLAB Function : MATLAB Function  TreatAsAtomicUnit=on
  room : Outport
  wires:
  MATLAB Function/1(roomOut) -> room/1

== system AreaCoverageTestHarness/Robot/thetaFilter ==
  thetaRaw : Inport
  Add : Sum  Inputs=+-
  Add1 : Sum
  Constant : Constant  Value=360
  Constant1 : Constant  Value=360
  Constant2 : Constant  Value=0
  Relational Operator : RelationalOperator  Operator=>  OutDataTypeStr=boolean
  Relational Operator1 : RelationalOperator  Operator=<  OutDataTypeStr=boolean
  Switch : Switch  Criteria=u2 > Threshold
  Switch1 : Switch  Criteria=u2 > Threshold
  thetaFiltered : Outport
  wires:
  thetaRaw/1 -> Switch1/3, Add/1, Add1/2, Relational Operator1/1, Relational Operator/1
  Constant/1 -> Add1/1, Relational Operator/2
  Relational Operator/1 -> Switch/2
  Constant1/1 -> Add/2
  Add/1 -> Switch/1
  Constant2/1 -> Relational Operator1/2
  Relational Operator1/1 -> Switch1/2
  Add1/1 -> Switch1/1
  Switch1/1 -> Switch/3
  Switch/1 -> thetaFiltered/1

== system AreaCoverageTestHarness/Robot/DetailedMap/createMap ==
  RoomV1 : Subsystem  VariantControl=Variant
  RoomV2 : Subsystem  VariantControl=Variant2
  RoomV3 : Subsystem  VariantControl=Variant3
  room : Outport

== system AreaCoverageTestHarness/Robot/EncoderTicksGenerator/Subsystem ==
  Enable : EnablePort  StatesWhenEnabling=reset
  Constant : Constant  Value=0.2
  Pulse Generator : DiscretePulseGenerator  PulseType=Time based  Period=.01  PulseWidth=50
  Scope : Scope
  Variable Time Delay : VariableTransportDelay  MaximumDelay=10
  EncoderPulses : Outport  OutputWhenDisabled=reset  InitialOutput=0
  wires:
  Pulse Generator/1 -> Variable Time Delay/1
  Constant/1 -> Variable Time Delay/2
  Variable Time Delay/1 -> Scope/1, EncoderPulses/1

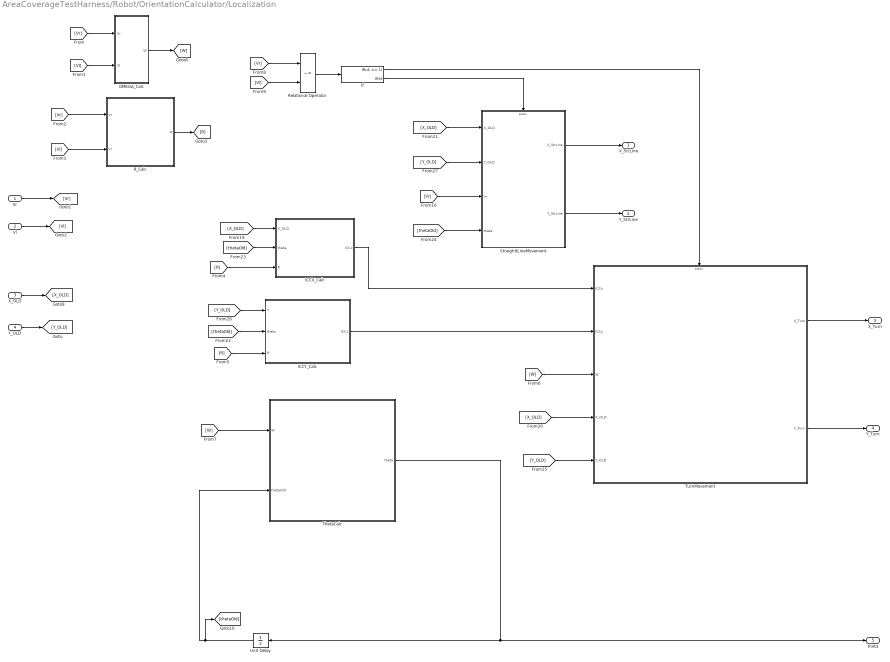
== system AreaCoverageTestHarness/Robot/OrientationCalculator/Localization ==
  Vr : Inport
  Vl : Inport  Port=2
  X_OLD : Inport  Port=3
  Y_OLD : Inport  Port=4
  ICCX_Calc : Subsystem
  ICCY_Calc : Subsystem
  If : If  IfExpression=u1 == 1
  OMEGA_Calc : Subsystem
  R_Calc : Subsystem
  Relational Operator : RelationalOperator  Operator=~=  OutDataTypeStr=boolean
  StraighltLineMovement : Subsystem  TreatAsAtomicUnit=on
  ThetaCalc : Subsystem
  TurnMovement : Subsystem
  Unit Delay : UnitDelay  InitialCondition=NORTH  SampleTime=-1
      settings: AttributesFormatString=%<InitialCondition>
  X_StrLine : Outport
  Y_StrLine : Outport  Port=2
  X_Turn : Outport  Port=3
  Y_Turn : Outport  Port=4
  theta : Outport  Port=5
  wires:
  [Y_OLD] -> TurnMovement/5(Y_OLD)
  [thetaOld] -> ICCY_Calc/2(theta)
  OMEGA_Calc/1(W) -> [W]
  ICCY_Calc/1(ICCy) -> TurnMovement/2(ICCy)
  ICCX_Calc/1(ICCx) -> TurnMovement/1(ICCx)
  [R] -> ICCY_Calc/3(R)
  [R] -> ICCX_Calc/3(R)
  R_Calc/1(R) -> [R]
  [Vl] -> R_Calc/2(Vl)
  [Vr] -> R_Calc/1(Vr)
  [Vl] -> OMEGA_Calc/2(Vl)
  [Vr] -> OMEGA_Calc/1(Vr)
  [Vr] -> StraighltLineMovement/3(Vr)
  If/2 -> StraighltLineMovement/Action
  If/1 -> TurnMovement/Action
  Relational Operator/1 -> If/1
  [Vr] -> Relational Operator/1
  [Vl] -> Relational Operator/2
  [W] -> TurnMovement/3(W)
  [X_OLD] -> TurnMovement/4(X_OLD)
  [X_OLD] -> ICCX_Calc/1(X_OLD)
  [thetaOld] -> ICCX_Calc/2(theta)
  [thetaOld] -> StraighltLineMovement/4(theta)
  StraighltLineMovement/2(Y_StrLine) -> Y_StrLine/1
  TurnMovement/1(X_Turn) -> X_Turn/1
  TurnMovement/2(Y_Turn) -> Y_Turn/1
  StraighltLineMovement/1(X_StrLine) -> X_StrLine/1
  [Y_OLD] -> StraighltLineMovement/2(Y_OLD)
  [Y_OLD] -> ICCY_Calc/1(Y)
  [X_OLD] -> StraighltLineMovement/1(X_OLD)
  Vr/1 -> [Vr]
  Vl/1 -> [Vl]
  Y_OLD/1 -> [Y_OLD]
  X_OLD/1 -> [X_OLD]
  Unit Delay/1 -> [thetaOld], ThetaCalc/2(thetaOld)
  ThetaCalc/1(theta) -> theta/1, Unit Delay/1
  [W] -> ThetaCalc/1(W)

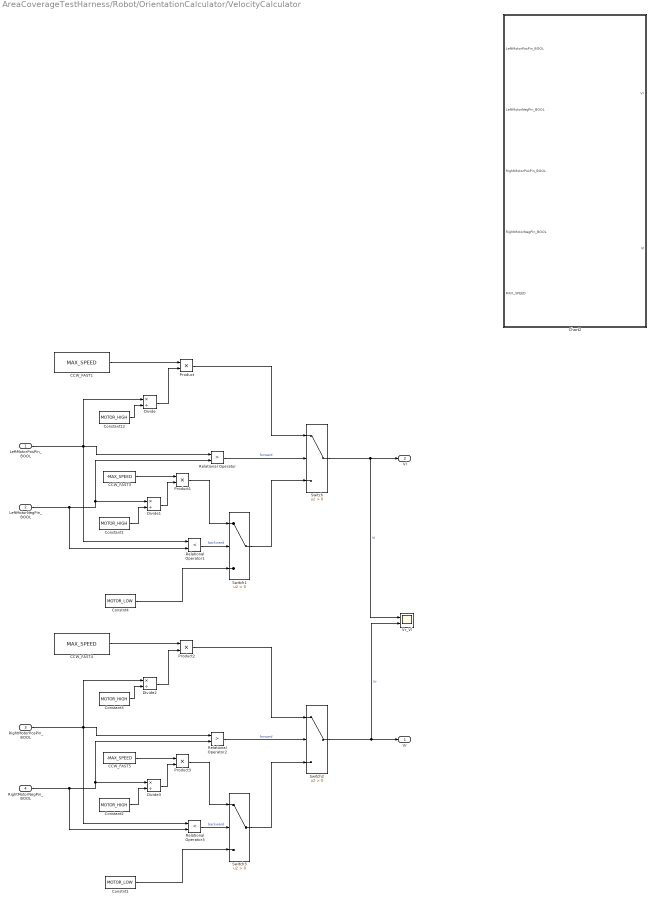
== system AreaCoverageTestHarness/Robot/OrientationCalculator/VelocityCalculator ==
  LeftMotorPosPin_BOOL : Inport
  LeftMotorNegPin_BOOL : Inport  Port=2
  RightMotorPosPin_BOOL : Inport  Port=3
  RightMotorNegPin_BOOL : Inport  Port=4
  CCW_FAST1 : Constant  Value=MAX_SPEED  OutDataTypeStr=int16  SampleTime=-1
  CCW_FAST3 : Constant  Value=-MAX_SPEED  OutDataTypeStr=int16  SampleTime=-1
  CCW_FAST4 : Constant  Value=MAX_SPEED  OutDataTypeStr=int16  SampleTime=-1
  CCW_FAST5 : Constant  Value=-MAX_SPEED  OutDataTypeStr=int16  SampleTime=-1
  Chart2 : Stateflow chart  TreatAsAtomicUnit=on
  Constant{1..3,12} (4 alike) : Constant  Value=MOTOR_HIGH
  Constnt1 : Constant  Value=MOTOR_LOW
  Constnt4 : Constant  Value=MOTOR_LOW
  Divide{,1..3} (4 alike) : Product  Inputs=*/
  Product{,1..3} (4 alike) : Product
  Relational Operator : RelationalOperator  Operator=>  OutDataTypeStr=boolean
  Relational Operator1 : RelationalOperator  Operator=<  OutDataTypeStr=boolean
  Relational Operator2 : RelationalOperator  Operator=>  OutDataTypeStr=boolean
  Relational Operator3 : RelationalOperator  Operator=<  OutDataTypeStr=boolean
  Switch{,1..3} (4 alike) : Switch  Criteria=u2 > Threshold
  Vr_Vl : Scope  NumInputPorts=2
  Vr : Outport
  Vl : Outport  Port=2
  wires:
  LeftMotorPosPin_BOOL/1 -> Divide/1, Relational Operator1/1, Relational Operator/1
  LeftMotorNegPin_BOOL/1 -> Relational Operator1/2, Relational Operator/2, Divide1/1
  Switch/1 -> Vr_Vl/1, Vl/1  "Vl"
  Relational Operator/1 -> Switch/2  "forward"
  Relational Operator1/1 -> Switch1/2  "backward"
  Constant12/1 -> Divide/2
  Divide/1 -> Product/2
  CCW_FAST1/1 -> Product/1
  Product/1 -> Switch/1
  Switch1/1 -> Switch/3
  Constant1/1 -> Divide1/2
  CCW_FAST3/1 -> Product1/1
  Divide1/1 -> Product1/2
  Product1/1 -> Switch1/1
  Constnt4/1 -> Switch1/3
  RightMotorPosPin_BOOL/1 -> Relational Operator2/1, Relational Operator3/1, Divide2/1
  RightMotorNegPin_BOOL/1 -> Divide3/1, Relational Operator2/2, Relational Operator3/2
  Relational Operator2/1 -> Switch2/2  "forward"
  Relational Operator3/1 -> Switch3/2  "backward"
  Constant3/1 -> Divide2/2
  Divide2/1 -> Product2/2
  CCW_FAST4/1 -> Product2/1
  Product2/1 -> Switch2/1
  Switch3/1 -> Switch2/3
  Constant2/1 -> Divide3/2
  CCW_FAST5/1 -> Product3/1
  Divide3/1 -> Product3/2
  Product3/1 -> Switch3/1
  Constnt1/1 -> Switch3/3
  Switch2/1 -> Vr_Vl/2, Vr/1  "Vr"

== system AreaCoverageTestHarness/Robot/RoomFilterSystem/StepCalc ==
  pos : Inport
  Chart : Stateflow chart  TreatAsAtomicUnit=on
  Data Type Conversion : DataTypeConversion  OutDataTypeStr=int32
  STEP_SIZE : Constant  Value=BLOCK_SIZE/4  OutDataTypeStr=int8
  Unit Delay : UnitDelay  SampleTime=-1
      settings: AttributesFormatString=%<InitialCondition>
  filteredStep : Outport
  wires:
  pos/1 -> Data Type Conversion/1
  Unit Delay/1 -> Chart/2(oldPos)
  Chart/1(step) -> filteredStep/1
  Data Type Conversion/1 -> Chart/1(pos), Unit Delay/1
  STEP_SIZE/1 -> Chart/3(STEP_SIZE)

== system AreaCoverageTestHarness/Robot/RoomFilterSystem/StepCalc1 ==
  pos : Inport
  Chart : Stateflow chart  TreatAsAtomicUnit=on
  Data Type Conversion : DataTypeConversion  OutDataTypeStr=int32
  STEP_SIZE : Constant  Value=BLOCK_SIZE/4  OutDataTypeStr=int8
  Unit Delay : UnitDelay  SampleTime=-1
      settings: AttributesFormatString=%<InitialCondition>
  filteredStep : Outport
  wires:
  STEP_SIZE/1 -> Chart/3(STEP_SIZE)
  Data Type Conversion/1 -> Unit Delay/1, Chart/1(pos)
  Chart/1(step) -> filteredStep/1
  Unit Delay/1 -> Chart/2(oldPos)
  pos/1 -> Data Type Conversion/1

== system AreaCoverageTestHarness/Robot/Subsystem1/OMEGA_Calc ==
  Vr : Inport
  Vl : Inport  Port=2
  Add : Sum  Inputs=+-
  Constant3 : Constant  Value=ROB_LENG
  Divide1 : Product  Inputs=*/
  W : Outport
  wires:
  Vl/1 -> Add/2
  Vr/1 -> Add/1
  Constant3/1 -> Divide1/2
  Divide1/1 -> W/1
  Add/1 -> Divide1/1

== system AreaCoverageTestHarness/Robot/Subsystem2/OMEGA_Calc ==
  Vr : Inport
  Vl : Inport  Port=2
  Add : Sum  Inputs=+-
  Constant3 : Constant  Value=ROB_LENG
  Divide1 : Product  Inputs=*/
  W : Outport
  wires:
  Add/1 -> Divide1/1
  Divide1/1 -> W/1
  Constant3/1 -> Divide1/2
  Vr/1 -> Add/1
  Vl/1 -> Add/2

== system AreaCoverageTestHarness/Robot/DetailedMap/createMap/RoomV1 ==
  Room_V1 : MATLAB Function  TreatAsAtomicUnit=on
  room : Outport
  wires:
  Room_V1/1(roomOut) -> room/1

== system AreaCoverageTestHarness/Robot/DetailedMap/createMap/RoomV2 ==
  Room_V2 : MATLAB Function  TreatAsAtomicUnit=on
  room : Outport
  wires:
  Room_V2/1(roomOut) -> room/1

== system AreaCoverageTestHarness/Robot/DetailedMap/createMap/RoomV3 ==
  Room_V3 : MATLAB Function  TreatAsAtomicUnit=on
  room : Outport
  wires:
  Room_V3/1(roomOut) -> room/1

== system AreaCoverageTestHarness/Robot/OrientationCalculator/Localization/ICCX_Calc ==
  X_OLD : Inport
  theta : Inport  Port=2
  R : Inport  Port=3
  FromDegreeToRad : Subsystem
  Product : Product
  ScopeTheta : Scope
  Subtract : Sum  Inputs=+-
  Trigonometric Function1 : Trigonometry
  ICCx : Outport
  wires:
  Product/1 -> Subtract/2
  X_OLD/1 -> Subtract/1
  FromDegreeToRad/1(Rad) -> Trigonometric Function1/1
  Subtract/1 -> ICCx/1
  theta/1 -> ScopeTheta/1, FromDegreeToRad/1(Deg)
  Trigonometric Function1/1 -> Product/2
  R/1 -> Product/1

== system AreaCoverageTestHarness/Robot/OrientationCalculator/Localization/ICCY_Calc ==
  Y : Inport
  theta : Inport  Port=2
  R : Inport  Port=3
  FromDegreeToRad : Subsystem
  Product : Product
  Subtract : Sum
  Trigonometric Function1 : Trigonometry  Operator=cos
  ICCy : Outport
  wires:
  Y/1 -> Subtract/1
  Trigonometric Function1/1 -> Product/2
  theta/1 -> FromDegreeToRad/1(Deg)
  Subtract/1 -> ICCy/1
  FromDegreeToRad/1(Rad) -> Trigonometric Function1/1
  Product/1 -> Subtract/2
  R/1 -> Product/1

== system AreaCoverageTestHarness/Robot/OrientationCalculator/Localization/OMEGA_Calc ==
  Vr : Inport
  Vl : Inport  Port=2
  Add : Sum  Inputs=+-
  Constant3 : Constant  Value=ROB_LENG  OutDataTypeStr=int16
  Divide1 : Product  Inputs=*/
  W : Outport
  wires:
  Vl/1 -> Add/2
  Vr/1 -> Add/1
  Constant3/1 -> Divide1/2
  Divide1/1 -> W/1
  Add/1 -> Divide1/1

== system AreaCoverageTestHarness/Robot/OrientationCalculator/Localization/R_Calc ==
  Vr : Inport
  Vl : Inport  Port=2
  If : If  NumInputs=2  IfExpression=u1 ~= u2  ShowElse=off
  If Action Subsystem1 : Subsystem  TreatAsAtomicUnit=on
  R : Outport
  wires:
  If/1 -> If Action Subsystem1/Action
  If Action Subsystem1/1(R) -> R/1
  Vr/1 -> If Action Subsystem1/1(Vr), If/1
  Vl/1 -> If/2, If Action Subsystem1/2(Vl)

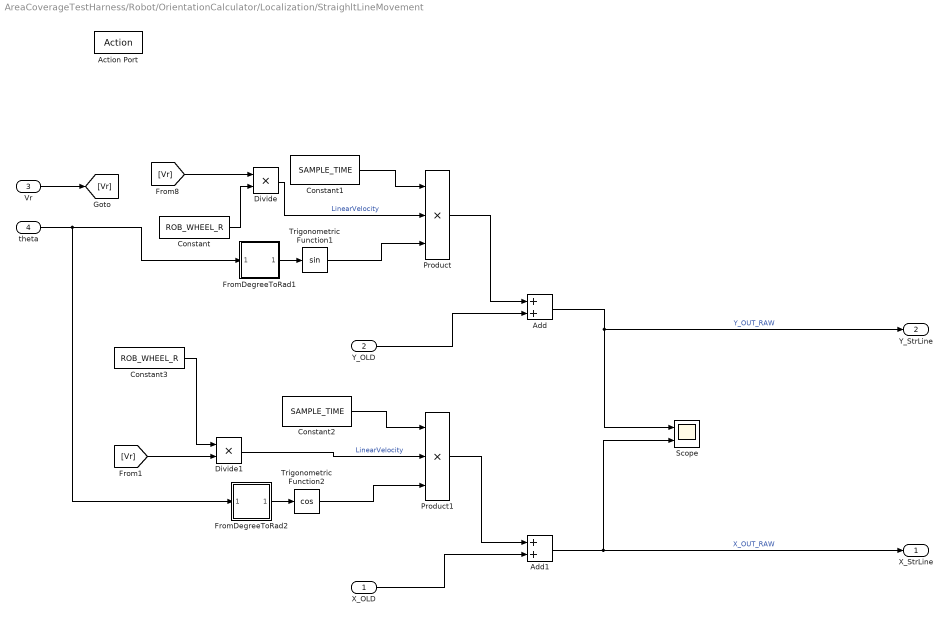
== system AreaCoverageTestHarness/Robot/OrientationCalculator/Localization/StraighltLineMovement ==
  X_OLD : Inport
  Y_OLD : Inport  Port=2
  Vr : Inport  Port=3
  theta : Inport  Port=4
  Action Port : ActionPort  ActionType=else
      settings: AttributesFormatString=%<InitializeStates>
  Add : Sum
  Add1 : Sum
  Constant : Constant  Value=ROB_WHEEL_R
  Constant1 : Constant  Value=SAMPLE_TIME  SampleTime=-1
  Constant2 : Constant  Value=SAMPLE_TIME  SampleTime=-1
  Constant3 : Constant  Value=ROB_WHEEL_R
  Divide : Product  Inputs=**
  Divide1 : Product  Inputs=**
  FromDegreeToRad1 : Subsystem
  FromDegreeToRad2 : Subsystem
  Product : Product  Inputs=3
  Product1 : Product  Inputs=3
  Scope : Scope  NumInputPorts=2
  Trigonometric Function1 : Trigonometry
  Trigonometric Function2 : Trigonometry  Operator=cos
  X_StrLine : Outport  InitialOutput=initXSim
      settings: AttributesFormatString=|
      | %<InitialOutput>
      | %<OutputWhenDisabled>
  Y_StrLine : Outport  Port=2  InitialOutput=initYSim
      settings: AttributesFormatString=|
      | %<InitialOutput>
      | %<OutputWhenDisabled>
  wires:
  FromDegreeToRad1/1(Rad) -> Trigonometric Function1/1
  Trigonometric Function1/1 -> Product/3
  Vr/1 -> [Vr]
  theta/1 -> FromDegreeToRad2/1(Deg), FromDegreeToRad1/1(Deg)
  Constant1/1 -> Product/1
  Y_OLD/1 -> Add/2
  Product/1 -> Add/1
  Add/1 -> Y_StrLine/1, Scope/1  "Y_OUT_RAW"
  FromDegreeToRad2/1(Rad) -> Trigonometric Function2/1
  Trigonometric Function2/1 -> Product1/3
  Constant2/1 -> Product1/1
  X_OLD/1 -> Add1/2
  Product1/1 -> Add1/1
  Add1/1 -> Scope/2, X_StrLine/1  "X_OUT_RAW"
  Constant/1 -> Divide/2
  [Vr] -> Divide/1
  Divide/1 -> Product/2  "LinearVelocity"
  [Vr] -> Divide1/2
  Constant3/1 -> Divide1/1
  Divide1/1 -> Product1/2  "LinearVelocity"

== system AreaCoverageTestHarness/Robot/OrientationCalculator/Localization/ThetaCalc ==
  W : Inport
  thetaOld : Inport  Port=2
  OrientationCalc : Subsystem
  thetaFilter : Subsystem
  theta : Outport
  wires:
  thetaFilter/1(thetaFiltered) -> theta/1
  W/1 -> OrientationCalc/1(W)
  OrientationCalc/1(Theta_OUT) -> thetaFilter/1(thetaRaw)
  thetaOld/1 -> OrientationCalc/2(theta_OLD)

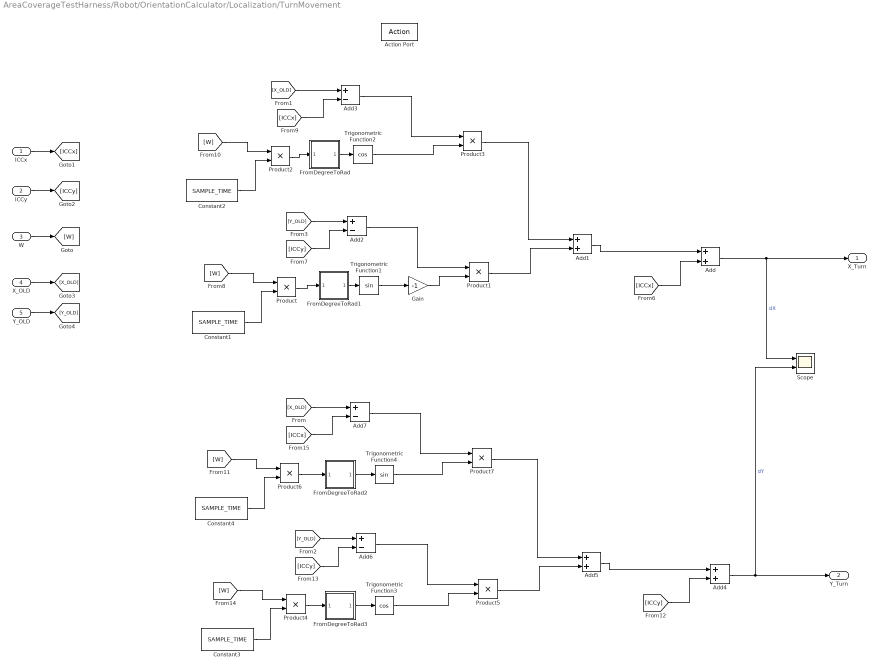
== system AreaCoverageTestHarness/Robot/OrientationCalculator/Localization/TurnMovement ==
  ICCx : Inport
  ICCy : Inport  Port=2
  W : Inport  Port=3
  X_OLD : Inport  Port=4
  Y_OLD : Inport  Port=5
  Action Port : ActionPort  ActionType=then
      settings: AttributesFormatString=%<InitializeStates>
  Add{,1,4..5} (4 alike) : Sum
  Add{2..3,6..7} (4 alike) : Sum  Inputs=+-
  Constant{1..4} (4 alike) : Constant  Value=SAMPLE_TIME  SampleTime=-1
  FromDegreeToRad : Subsystem
  FromDegreeToRad1 : Subsystem
  FromDegreeToRad2 : Subsystem
  FromDegreeToRad3 : Subsystem
  Gain : Gain  Gain=-1
  Product{,1..7} (8 alike) : Product
  Scope : Scope  NumInputPorts=2
  Trigonometric Function1 : Trigonometry
  Trigonometric Function2 : Trigonometry  Operator=cos
  Trigonometric Function3 : Trigonometry  Operator=cos
  Trigonometric Function4 : Trigonometry
  X_Turn : Outport  InitialOutput=initXSim
      settings: AttributesFormatString=|
      | %<InitialOutput>
      | %<OutputWhenDisabled>
  Y_Turn : Outport  Port=2  InitialOutput=initYSim
      settings: AttributesFormatString=|
      | %<InitialOutput>
      | %<OutputWhenDisabled>
  wires:
  [W] -> Product/1
  Gain/1 -> Product1/2
  [ICCx] -> Add/2
  Add2/1 -> Product1/1
  Add1/1 -> Add/1
  Product2/1 -> FromDegreeToRad/1(Deg)
  Product1/1 -> Add1/2
  Constant1/1 -> Product/2
  Add3/1 -> Product3/1
  Add/1 -> Scope/1, X_Turn/1  "dX"
  Product/1 -> FromDegreeToRad1/1(Deg)
  Trigonometric Function1/1 -> Gain/1
  [ICCy] -> Add2/2
  Constant2/1 -> Product2/2
  Trigonometric Function2/1 -> Product3/2
  [ICCx] -> Add3/2
  [W] -> Product2/1
  Product3/1 -> Add1/1
  Add6/1 -> Product5/1
  [ICCy] -> Add4/2
  Product5/1 -> Add5/2
  Product7/1 -> Add5/1
  Add7/1 -> Product7/1
  Product6/1 -> FromDegreeToRad2/1(Deg)
  Trigonometric Function3/1 -> Product5/2
  Add5/1 -> Add4/1
  Trigonometric Function4/1 -> Product7/2
  [W] -> Product4/1
  Add4/1 -> Scope/2, Y_Turn/1  "dY"
  [ICCy] -> Add6/2
  [ICCx] -> Add7/2
  Constant3/1 -> Product4/2
  Product4/1 -> FromDegreeToRad3/1(Deg)
  [W] -> Product6/1
  Constant4/1 -> Product6/2
  W/1 -> [W]
  ICCx/1 -> [ICCx]
  ICCy/1 -> [ICCy]
  FromDegreeToRad/1(Rad) -> Trigonometric Function2/1
  FromDegreeToRad1/1(Rad) -> Trigonometric Function1/1
  FromDegreeToRad2/1(Rad) -> Trigonometric Function4/1
  FromDegreeToRad3/1(Rad) -> Trigonometric Function3/1
  X_OLD/1 -> [X_OLD]
  [X_OLD] -> Add7/1
  [X_OLD] -> Add3/1
  Y_OLD/1 -> [Y_OLD]
  [Y_OLD] -> Add6/1
  [Y_OLD] -> Add2/1

== system AreaCoverageTestHarness/Robot/OrientationCalculator/Localization/ICCX_Calc/FromDegreeToRad ==
  Deg : Inport
  Constant1 : Constant  Value=pi
  Constant2 : Constant  Value=180
  Divide : Product  Inputs=*/
  Product : Product
  Rad : Outport
  wires:
  Divide/1 -> Product/1
  Deg/1 -> Product/2
  Constant1/1 -> Divide/1
  Product/1 -> Rad/1
  Constant2/1 -> Divide/2

== system AreaCoverageTestHarness/Robot/OrientationCalculator/Localization/ICCY_Calc/FromDegreeToRad ==
  Deg : Inport
  Constant1 : Constant  Value=pi
  Constant2 : Constant  Value=180
  Divide : Product  Inputs=*/
  Product : Product
  Rad : Outport
  wires:
  Divide/1 -> Product/1
  Deg/1 -> Product/2
  Constant1/1 -> Divide/1
  Product/1 -> Rad/1
  Constant2/1 -> Divide/2

== system AreaCoverageTestHarness/Robot/OrientationCalculator/Localization/R_Calc/If Action Subsystem1 ==
  Vr : Inport
  Vl : Inport  Port=2
  Action Port : ActionPort  InitializeStates=reset  ActionType=then
      settings: AttributesFormatString=%<InitializeStates>
  Add : Sum
  Add1 : Sum  Inputs=+-
  Constant3 : Constant  Value=ROB_LENG
  Constant4 : Constant  Value=2  OutDataTypeStr=int16
  Divide1 : Product  Inputs=*/
  Divide2 : Product  Inputs=*/
  Product1 : Product
  Vr1 : InportShadow
  R : Outport  OutputWhenDisabled=reset  InitialOutput=0
      settings: AttributesFormatString=|
      | Mode: %<OutputWhenDisabled>
      | InitialOuput: %<InitialOutput>
  wires:
  Vr1/1 -> Add1/1
  Vr/1 -> Add/1
  Add1/1 -> Divide2/2
  Add/1 -> Divide2/1
  Divide1/1 -> Product1/2
  Divide2/1 -> Product1/1
  Constant3/1 -> Divide1/1
  Product1/1 -> R/1
  Vl/1 -> Add1/2, Add/2
  Constant4/1 -> Divide1/2

== system AreaCoverageTestHarness/Robot/OrientationCalculator/Localization/StraighltLineMovement/FromDegreeToRad1 ==
  Deg : Inport
  Constant1 : Constant  Value=pi
  Constant2 : Constant  Value=180
  Divide : Product  Inputs=*/
  Product : Product
  Rad : Outport
  wires:
  Constant2/1 -> Divide/2
  Product/1 -> Rad/1
  Constant1/1 -> Divide/1
  Deg/1 -> Product/2
  Divide/1 -> Product/1

== system AreaCoverageTestHarness/Robot/OrientationCalculator/Localization/StraighltLineMovement/FromDegreeToRad2 ==
  Deg : Inport
  Constant1 : Constant  Value=pi
  Constant2 : Constant  Value=180
  Divide : Product  Inputs=*/
  Product : Product
  Rad : Outport
  wires:
  Divide/1 -> Product/1
  Deg/1 -> Product/2
  Constant1/1 -> Divide/1
  Product/1 -> Rad/1
  Constant2/1 -> Divide/2

== system AreaCoverageTestHarness/Robot/OrientationCalculator/Localization/ThetaCalc/OrientationCalc ==
  W : Inport
  theta_OLD : Inport  Port=2
  Add : Sum
  Constant4 : Constant  Value=SAMPLE_TIME  SampleTime=-1
  Product : Product
  Theta_OUT : Outport
  wires:
  theta_OLD/1 -> Add/2
  Constant4/1 -> Product/2
  W/1 -> Product/1
  Add/1 -> Theta_OUT/1
  Product/1 -> Add/1

== system AreaCoverageTestHarness/Robot/OrientationCalculator/Localization/ThetaCalc/thetaFilter ==
  thetaRaw : Inport
  Add : Sum  Inputs=+-
  Add1 : Sum
  Constant : Constant  Value=360
  Constant1 : Constant  Value=360
  Constant2 : Constant  Value=0
  Relational Operator : RelationalOperator  Operator=>  OutDataTypeStr=boolean
  Relational Operator1 : RelationalOperator  Operator=<  OutDataTypeStr=boolean
  Switch : Switch  Criteria=u2 > Threshold
  Switch1 : Switch  Criteria=u2 > Threshold
  Theta : Scope
  thetaFiltered : Outport
  wires:
  thetaRaw/1 -> Switch1/3, Add/1, Add1/2, Relational Operator1/1, Relational Operator/1
  Constant/1 -> Add1/1, Relational Operator/2
  Relational Operator/1 -> Switch/2
  Constant1/1 -> Add/2
  Add/1 -> Switch/1
  Constant2/1 -> Relational Operator1/2
  Relational Operator1/1 -> Switch1/2
  Add1/1 -> Switch1/1
  Switch1/1 -> Switch/3
  Switch/1 -> Theta/1, thetaFiltered/1

== system AreaCoverageTestHarness/Robot/OrientationCalculator/Localization/TurnMovement/FromDegreeToRad ==
  Deg : Inport
  Constant1 : Constant  Value=pi
  Constant2 : Constant  Value=180
  Divide : Product  Inputs=*/
  Product : Product
  Rad : Outport
  wires:
  Divide/1 -> Product/1
  Deg/1 -> Product/2
  Constant1/1 -> Divide/1
  Product/1 -> Rad/1
  Constant2/1 -> Divide/2

== system AreaCoverageTestHarness/Robot/OrientationCalculator/Localization/TurnMovement/FromDegreeToRad1 ==
  Deg : Inport
  Constant1 : Constant  Value=pi
  Constant2 : Constant  Value=180
  Divide : Product  Inputs=*/
  Product : Product
  Rad : Outport
  wires:
  Constant2/1 -> Divide/2
  Product/1 -> Rad/1
  Constant1/1 -> Divide/1
  Deg/1 -> Product/2
  Divide/1 -> Product/1

== system AreaCoverageTestHarness/Robot/OrientationCalculator/Localization/TurnMovement/FromDegreeToRad2 ==
  Deg : Inport
  Constant1 : Constant  Value=pi
  Constant2 : Constant  Value=180
  Divide : Product  Inputs=*/
  Product : Product
  Rad : Outport
  wires:
  Divide/1 -> Product/1
  Deg/1 -> Product/2
  Constant1/1 -> Divide/1
  Product/1 -> Rad/1
  Constant2/1 -> Divide/2

== system AreaCoverageTestHarness/Robot/OrientationCalculator/Localization/TurnMovement/FromDegreeToRad3 ==
  Deg : Inport
  Constant1 : Constant  Value=pi
  Constant2 : Constant  Value=180
  Divide : Product  Inputs=*/
  Product : Product
  Rad : Outport
  wires:
  Constant2/1 -> Divide/2
  Product/1 -> Rad/1
  Constant1/1 -> Divide/1
  Deg/1 -> Product/2
  Divide/1 -> Product/1
